simulink model "EmbeddedMatlabFunction"  (Simulink 7.4)
settings: Solver=ode45  StartTime=0.0  StopTime=10.0  RelTol=1e-3
settings Model: Creator=dread  LastModifiedBy=dread

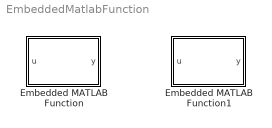
== system EmbeddedMatlabFunction ==
  Embedded MATLAB Function : Stateflow chart
  Embedded MATLAB Function1 : Stateflow chart

== matlab function Embedded MATLAB Function1 ==
  data: u input uint8; y output uint8
function y = fcn(u)
%#eml

y = u;

== matlab function Embedded MATLAB Function ==
  data: u input uint8; y output uint8
function y = fcn(u)
%#eml

y = u;
